simulink model "Kalman_Filter"  (R2023a)
settings: Solver=VariableStepAuto  StartTime=0.0  StopTime=3  RelTol=1e-3
settings Model: Creator=Vims  LastModifiedBy=Vims

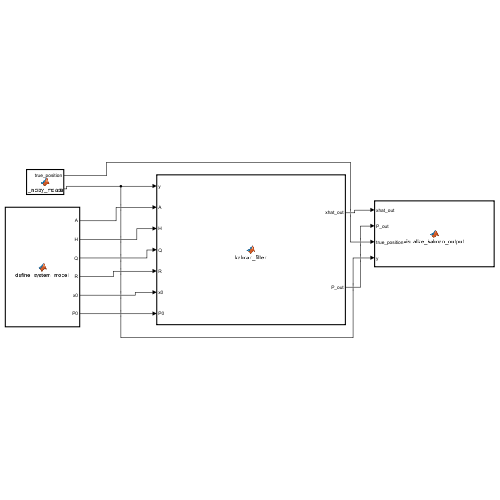
[thumbnail: Simulink's stored preview of the top-level diagram]
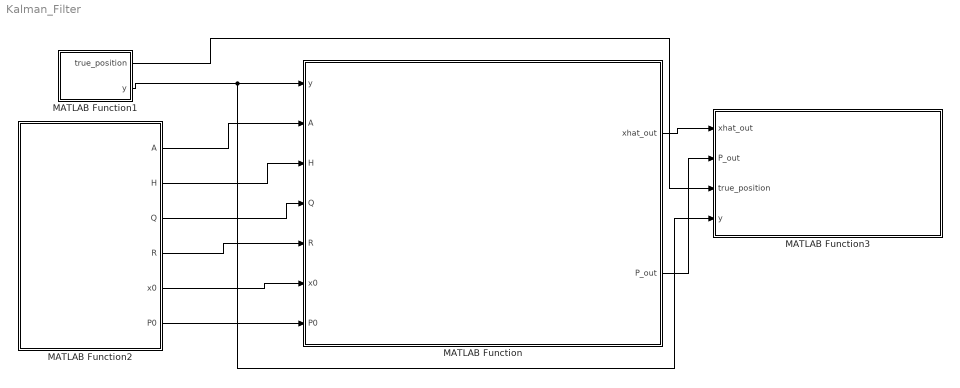
== system Kalman_Filter ==
  MATLAB Function : MATLAB Function  TreatAsAtomicUnit=on
  MATLAB Function1 : MATLAB Function  TreatAsAtomicUnit=on
  MATLAB Function2 : MATLAB Function  TreatAsAtomicUnit=on
  MATLAB Function3 : MATLAB Function  TreatAsAtomicUnit=on
  wires:
  MATLAB Function2/1(A) -> MATLAB Function/2(A)
  MATLAB Function2/2(H) -> MATLAB Function/3(H)
  MATLAB Function2/3(Q) -> MATLAB Function/4(Q)
  MATLAB Function2/4(R) -> MATLAB Function/5(R)
  MATLAB Function2/5(x0) -> MATLAB Function/6(x0)
  MATLAB Function2/6(P0) -> MATLAB Function/7(P0)
  MATLAB Function/1(xhat_out) -> MATLAB Function3/1(xhat_out)
  MATLAB Function/2(P_out) -> MATLAB Function3/2(P_out)
  MATLAB Function1/2(y) -> MATLAB Function3/4(y), MATLAB Function/1(y)
  MATLAB Function1/1(true_position) -> MATLAB Function3/3(true_position)

== matlab function Kalman_Filter/MATLAB Function1 ==
  data: true_position output; y output
function [true_position, y] = generate_noisy_measurements()
    % True sinusoidal trajectory parameters
    time_steps = 50;
    amplitude = 10;
    frequency = 0.2; % Adjust for desired oscillations 
    phase_shift = 0; % Adjust phase shift if needed

    % Generate time vector
    t = 0:time_steps-1; 

    % Generate the 'true' sinusoidal trajectory
    true_position = amplitude * sin(2*pi*frequency*t + phase_shift); 

    % Measurement noise parameters
    measurement_std_dev = 2; 

    % Generate noisy measurements
    noise = measurement_std_dev * randn(size(true_position)); 
    y = true_position + noise;
end

== matlab function Kalman_Filter/MATLAB Function ==
  data: y input; xhat_out output; A input; H input; Q input; R input; x0 input; P0 input; P_out output
function [xhat_out, P_out] = kalman_filter(y, A, H, Q, R, x0, P0)
    % Initialize state and covariance
    xhat = x0;
    P = P0;

    % Pre-allocation for efficiency 
    xhat_out = zeros(size(x0, 1), length(y));  % Rows matching x0, columns matching y
    % P_out = zeros(size(P0), length(y));      % Dimensions of P0, columns matching y
[num_rows, num_cols] = size(P0);
P_out = zeros(num_rows, num_cols, length(y)); 

    % Kalman filter loop
    for k = 1:length(y)
        % Prediction
        xhat_pred = A * xhat;
        P_pred = A * P * A' + Q;

        % Update
        K = P_pred * H' / (H * P_pred * H' + R);
        xhat = xhat_pred + K * (y(k) - H * xhat_pred);
        P = (eye(size(K*H)) - K * H) * P_pred;

        % Store the results
        xhat_out(:,k) = xhat; 
        P_out(:,:,k) = P; 

    end
end


% y: A vector of measurements.
% A: The state transition matrix.
% H: The measurement matrix.
% Q: The process noise covariance.
% R: The measurement noise covariance.
% x0: Initial state estimate.
% P0: Initial state covariance estimate.


% % System Parameters (assuming constant velocity model)
% dt = 0.1; % Time step
% A = [1 dt; 0 1]; 
% H = [1 0];
% Q = [0.01 0; 0 0.01]; 
% R = 0.5; 
% x0 = [0; 0]; % Initial state (position, velocity) 
% P0 = eye(2);
% 
% % Simulate measurements... 
% 
% % Run Kalman Filter
% [xhat_out, P_out] = kalman_filter(y, A, H, Q, R, x0, P0);

== matlab function Kalman_Filter/MATLAB Function2 ==
  data: A output; H output; Q output; R output; x0 output; P0 output
function [A, H, Q, R, x0, P0] = define_system_model()
    % System Parameters (assuming constant velocity model)
    dt = 0.1; % Time step

    % Define matrices
    A = [1 dt; 0 1]; 
    H = [1 0];
    Q = [0.01 0; 0 0.01]; 
    R = 0.5; 

    % Initial Conditions
    x0 = [0; 0]; % Initial state (position, velocity) 
    P0 = eye(2);

end

== matlab function Kalman_Filter/MATLAB Function3 ==
  data: xhat_out input; P_out input; true_position input; y input
function visualize_kalman_output(xhat_out, P_out, true_position, y) 
    % Initialize arrays to store data from all iterations
    all_xhat_pos = []; 
    all_errors = [];

    % Extract data from each iteration
    for i = 1:size(xhat_out, 2) 
        % Store current estimated position
        all_xhat_pos = [all_xhat_pos xhat_out(1, i)];

        % Calculate estimation error (optional)
        if nargin > 3 
            error = xhat_out(1, i) - true_position(i);
            all_errors = [all_errors error];
        end
    end

    % Plot everything in one figure after the loop
    figure; 
    hold on; 

    % Plot estimated positions 
    plot(all_xhat_pos, 'g', 'LineWidth', 2);  

    % Include true positions (if available)
    if nargin > 3
        plot(true_position, 'b', 'LineWidth', 2); 
    end

    % Plot measurements 
    plot(y, 'r.', 'MarkerSize', 15); 

    % Labels, title, and legend
    xlabel('Time Step');
    ylabel('Position');
    title('Kalman Filter Output');
    if nargin > 3
        legend('Kalman Estimate', 'True Position', 'Measurements');
    else
        legend('Kalman Estimate', 'Measurements'); 
    end

    % (Optional) Plot estimation error 
    if nargin > 3
        plot(all_errors, 'k--', 'LineWidth', 1.5); 
        legend('Kalman Estimate', 'True Position', 'Measurements', 'Error'); 
    end
end
